simulink model "fx_v_TxRx_n7_imprv_final"  (R2020a)
settings: Solver=VariableStepAuto  StartTime=0.0  StopTime=500  RelTol=1e-3
undefined symbols (not defined in the file or in its folder): A, N
libraries: xbsIndex_r4 x8, dspsrcs4 x1, JTAGRuntimeCosim_r4 x1
settings Model: Creator=RaviM  LastModifiedBy=RaviM

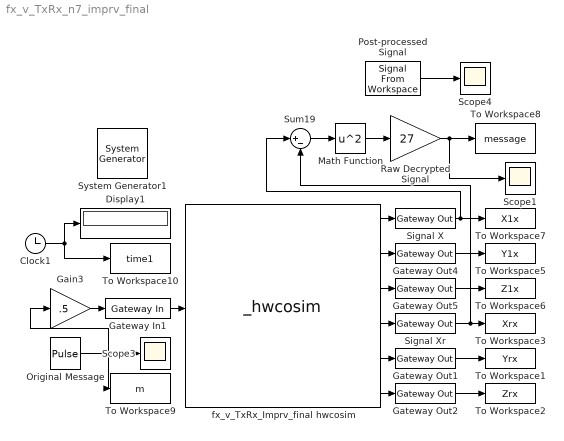
== system fx_v_TxRx_n7_imprv_final ==
  " System Generator1" : xbsIndex_r4/ System Generator  Tag=genX  xilinxfamily=artix7  part=xc7a100t  speed=-1  package=csg324  synthesis_tool=Vivado  clock_wrapper=Clock Enables  directory=C:/CSULB/test_int_n7_3  proj_type=Vivado  Synth_file=Vivado Synthesis Defaults  Impl_file=Vivado Implementation Defaults  testbench=off  simulink_period=1/100  sysclk_period=100  dcm_input_clock_period=10  incr_netlist=off  trim_vbits=Everywhere in SubSystem  dbl_ovrd=According to Block Masks  core_generation=According to Block Masks  run_coregen=off  deprecated_control=off  eval_field=0  block_type=sysgen
  Clock1 : Clock
  Display1 : Display
      settings: Decimation=5
  Gain3 : Gain  Gain=.5
  Gateway In1 : xbsIndex_r4/Gateway In  gui_display_data_type=Fixed-point  arith_type="Signed  (2's comp)"  n_bits=16  bin_pt=14  preci_type=Single  exp_width=8  frac_width=24  rows=1  columns=1  quantization="Round  (unbiased: +/- Inf)"  overflow=Saturate  period=1  UseAsADC=off  ADCChannel='1'  interface=None  automatic_assignment=on  address_offset=hex2dec('00')  intf_name=''  intf_description=''  default_value=0  timing_constraint=None  locs_specified=off  LOCs={}  io_standard={}  inherit_from_input=off  hdl_port=on  dbl_ovrd=off  block_type=gatewayin
  Gateway Out{1..2,4..5} (4 alike) : xbsIndex_r4/Gateway Out  inherit_from_input=off  hdl_port=on  rows=1  columns=1  UseAsDAC=off  DACChannel='1'  interface=None  automatic_assignment=on  address_offset=hex2dec('00')  intf_name=''  intf_description=''  timing_constraint=None  locs_specified=off  LOCs={}  io_standard={}  block_type=gatewayout
  Math Function : Math  Operator=square  SignedPower=on  SaturateOnIntegerOverflow=on
  Original Message : DiscretePulseGenerator  PulseType=Time based  Amplitude=5  Period=100  PulseWidth=50  PhaseDelay=50
  Post-processed Signal : dspsrcs4/Signal From Workspace  X=decrypted  Ts=0.01  nsamps=10  OutputAfterFinalValue=Setting to zero  ignoreOrWarnInputAndFrameLengths=off  OutputFrames=off
  Raw Decrypted Signal : Gain  Gain=27
  Scope1 : Scope
  Scope3 : Scope
  Scope4 : Scope
  Signal X : xbsIndex_r4/Gateway Out  inherit_from_input=off  hdl_port=on  rows=1  columns=1  UseAsDAC=off  DACChannel='1'  interface=None  automatic_assignment=on  address_offset=hex2dec('00')  intf_name=''  intf_description=''  timing_constraint=None  locs_specified=off  LOCs={}  io_standard={}  block_type=gatewayout
  Signal Xr : xbsIndex_r4/Gateway Out  inherit_from_input=off  hdl_port=on  rows=1  columns=1  UseAsDAC=off  DACChannel='1'  interface=None  automatic_assignment=on  address_offset=hex2dec('00')  intf_name=''  intf_description=''  timing_constraint=None  locs_specified=off  LOCs={}  io_standard={}  block_type=gatewayout
  Sum19 : Sum  Inputs=|+-
  To Workspace1 : ToWorkspace  VariableName=Yrx  SaveFormat=Timeseries  SampleTime=-1
  To Workspace10 : ToWorkspace  VariableName=time1  SampleTime=-1
  To Workspace2 : ToWorkspace  VariableName=Zrx  SaveFormat=Timeseries  SampleTime=-1
  To Workspace3 : ToWorkspace  VariableName=Xrx  SaveFormat=Timeseries  SampleTime=-1
  To Workspace5 : ToWorkspace  VariableName=Y1x  SaveFormat=Timeseries  SampleTime=-1
  To Workspace6 : ToWorkspace  VariableName=Z1x  SaveFormat=Timeseries  SampleTime=-1
  To Workspace7 : ToWorkspace  VariableName=X1x  SaveFormat=Timeseries  SampleTime=-1
  To Workspace8 : ToWorkspace  VariableName=message  SampleTime=-1
  To Workspace9 : ToWorkspace  VariableName=m  SampleTime=-1
  fx_v_TxRx_Imprv_final hwcosim : JTAGRuntimeCosim_r4/_hwcosim  clkSrc=Single Stepped  hasCombinationalPath=on  bitfileName=C:\CSULB\Final\fx_v_txrx_imprv_final.bit  skipConfig=off  dispPartInfo=off  useZynqReconfigScript=on  cable=Auto Detect  speed=N/A  cablePort=N/A  cableLocation=Local  shareCable=off  design_xtable=|  engineDll=JTAGCosimEngine.dll  cableWaitTime=10  bscanPos=-1  IRLengths=[]  useWaitBox=1  hasBufgmux=on  Scheme=Cosim  useCmdProc=1  hasProc=0  useImpact=0  printLogFile=0  userChain=2  block_type=jtagcosim
      | {
      |     'clkWrapper' => 'fx_v_txrx_imprv_final',
      |     'burstMode' => false,
      |     'burstFifoDepth' => '1024',
      |     'shared_memories' => {},
      |     'clocksGcd' => 1,
      |     'device' => {
      |       'family' => 'artix7',
      |       'part' => 'xc7a100t',
      |       'package' => 'csg324',
      |       'speed' => '-1',
      |     },
      |     'ports' => {
      |       'gateway_in1' => {
      |         'direction' => 'in',
      |         'width' => 16,
      |         'name' => 'gateway_in1',
      |         'period' => 100,
      |         'icon_text' => 'Gateway In1',
      |         'type' => 'Fix_16_14',
      |         'arithmetic_type' => 'xlSigned',
      |         'dat_file' => 'fx_v_txrx_imprv_final_gateway_in1.dat',
      |         'bin_pt' => 14,
      |         'addr_offset' => 0,
      |         'bd_port_index' => 0,
      |       },
      |       'gateway_out' => {
      |         'direction' => 'out',
      |         'width' => 32,
      |         'name' => 'gateway_out',
      |         'period' => 1,
      |         'icon_text' => 'Gateway Out',
      |         'type' => 'Fix_32_24',
      |         'arithmetic_type' => 'xlSigned',
      |         'dat_file' => 'fx_v_txrx_imprv_final_gateway_out.dat',
      |         'bin_pt' => 24,
      |         'addr_offset' => 4,
      |         'bd_port_index' => 0,
      |       },
      |       'gateway_out1' => {
      |         'direction' => 'out',
      |         'width' => 32,
      |         'name' => 'gateway_out1',
      |         'period' => 1,
      |         'icon_text' => 'Gateway Out1',
      |         'type' => 'Fix_32_24',
      |         'arithmetic_type' => 'xlSigned',
      |         'dat_file' => 'fx_v_txrx_imprv_final_gateway_out1.dat',
      |         'bin_pt' => 24,
      |         'addr_offset' => 8,
      |         'bd_port_index' => 1,
      |       },
      |       'gateway_out2' => {
      |         'direction' => 'out',
      |         'width' => 32,
      |         'name' => 'gateway_out2',
      |         'period' => 1,
      |         'icon_text' => 'Gateway Out2',
      |         'type' => 'Fix_32_24',
      |         'arithmetic_type' => 'xlSigned',
      |         'dat_file' => 'fx_v_txrx_imprv_final_gateway_out2.dat',
      |         'bin_pt' => 24,
      |         'addr_offset' => 12,
      |         'bd_port_index' => 2,
      |       },
      |       'gateway_out3' => {
      |         'direction' => 'out',
      |         'width' => 32,
      |         'name' => 'gateway_out3',
      |         'period' => 1,
      |         'icon_text' => 'Gateway Out3',
      |         'type' => 'Fix_32_24',
      |         'arithmetic_type' => 'xlSigned',
      |         'dat_file' => 'fx_v_txrx_imprv_final_gateway_out3.dat',
      |         'bin_pt' => 24,
      |         'addr_offset' => 16,
      |         'bd_port_index' => 3,
      |       },
      |       'gateway_out4' => {
      |         'direction' => 'out',
      |         'width' => 32,
      |         'name' => 'gateway_out4',
      |         'period' => 1,
      |         'icon_text' => 'Gateway Out4',
      |         'type' => 'Fix_32_24',
      |         'arithmetic_type' => 'xlSigned',
      |         'dat_file' => 'fx_v_txrx_imprv_final_gateway_out4.dat',
      |         'bin_pt' => 24,
      |         'addr_offset' => 20,
      |         'bd_port_index' => 4,
      |       },
      |       'gateway_out5' => {
      |         'direction' => 'out',
      |         'width' => 32,
      |         'name' => 'gateway_out5',
      |         'period' => 1,
      |         'icon_text' => 'Gateway Out5',
      |         'type' => 'Fix_32_24',
      |         'arithmetic_type' => 'xlSigned',
      |         'dat_file' => 'fx_v_txrx_imprv_final_gateway_out5.dat',
      |         'bin_pt' => 24,
      |         'addr_offset' => 24,
      |         'bd_port_index' => 5,
      |       },
      |     },
      |   }
  wires:
  fx_v_TxRx_Imprv_final hwcosim/5 -> Gateway Out1/1
  Math Function/1 -> Raw Decrypted Signal/1
  Gain3/1 -> Gateway In1/1
  fx_v_TxRx_Imprv_final hwcosim/6 -> Gateway Out2/1
  fx_v_TxRx_Imprv_final hwcosim/4 -> Signal Xr/1
  Signal X/1 -> Sum19/1, To Workspace7/1
  Gateway Out5/1 -> To Workspace6/1
  Gateway Out4/1 -> To Workspace5/1
  Original Message/1 -> To Workspace9/1, Scope3/1, Gain3/1
  Raw Decrypted Signal/1 -> Scope1/1, To Workspace8/1
  Gateway In1/1 -> fx_v_TxRx_Imprv_final hwcosim/1
  fx_v_TxRx_Imprv_final hwcosim/3 -> Gateway Out5/1
  Sum19/1 -> Math Function/1
  fx_v_TxRx_Imprv_final hwcosim/2 -> Gateway Out4/1
  Signal Xr/1 -> To Workspace3/1, Sum19/2
  fx_v_TxRx_Imprv_final hwcosim/1 -> Signal X/1
  Gateway Out2/1 -> To Workspace2/1
  Gateway Out1/1 -> To Workspace1/1
  Clock1/1 -> To Workspace10/1, Display1/1
  Post-processed Signal/1 -> Scope4/1
